simulink model "Simulation_3DOF02Testing"  (R2024a)
settings: Solver=ode4  StartTime=initial_time  StopTime=final_time  FixedStep=timestep  RelTol=1e-3
values from neighbouring files (symbols this model uses):
  alphaArray = [-30, -25, -20, -15, -10, -5, 0, 5, 10, 15, 20, 25, 30]    [Constants_3DOF.m]
  altitudeArray = [0, 1000, 2000, 3000, 4000, 5000, 6000, 7000, 8000, 9000, 10000, 15000, 20000,      25000, 30000, 35000, 40000, 45000, 50000, 55000, 60000]    [Constants_3DOF.m]
  cD_3DArray = zeros(numAoAs, numMachs, numAltitudes)    [Constants_3DOF.m]
  cL_3DArray = zeros(numAoAs, numMachs, numAltitudes)    [Constants_3DOF.m]
  flight_path_angle_0 = flight_path_angle_0 * (pi / 180)    (= 0.0523598775598)    [Constants_3DOF.m]
  heading_angle_0 = heading_angle_0 * (pi/180)    (= 0.349065850399)    [Constants_3DOF.m]
  height_0 = 35 * 10^3    (= 35000)    [Constants_3DOF.m]
  heightsList = usAtmosphere.Z    [Constants_3DOF.m]
  latitude_0 = latitude_0 * (pi/180)    (= 0.680503875353)    [Constants_3DOF.m]
  longitude_0 = longitude_0 * (pi/180)    (= -1.26396744429)    [Constants_3DOF.m]
  machArray = [0.5, 1.0, 1.5, 2.0, 2.5, 3.0, 3.5, 4.0, 4.5, 5.0, 5.5, 6.0, 6.5, 7.0, 7.5, 8.0,      8.5, 9.0, 9.5, 10.0]    [Constants_3DOF.m]
  mass = 161.5    [Constants_3DOF.m]
  omega_earth = 7.2921159 * 10^-5    (= 7.2921159e-05)    [Constants_3DOF.m]
  optimalAoA = zeros(numMachs, numAltitudes)    [Constants_3DOF.m]
  r_earth = 6371.0088 * 10^3    (= 6371008.8)    [Constants_3DOF.m]
  range_0 = 0    [Constants_3DOF.m]
  range_to_go_0 = 11112 * 10^3    (= 11112000)    [Constants_3DOF.m]
  rhoList = usAtmosphere.x_    [Constants_3DOF.m]
  speed_0 = 1500    [Constants_3DOF.m]
  temperatureList = usAtmosphere.T    [Constants_3DOF.m]
  wing_area = 0.079813    [Constants_3DOF.m]
libraries: simulink_extras x5
settings Model: Creator=641893  LastModifiedBy=641893

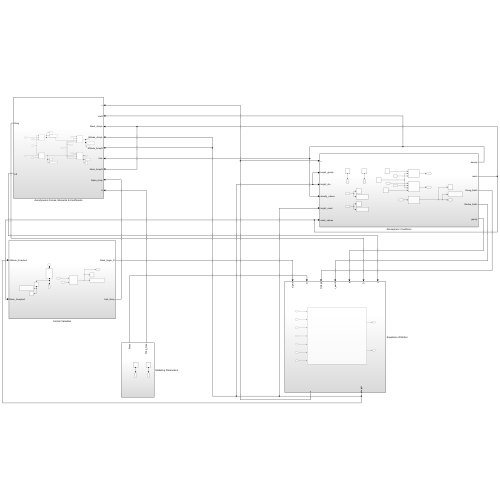
[thumbnail: Simulink's stored preview of the top-level diagram]
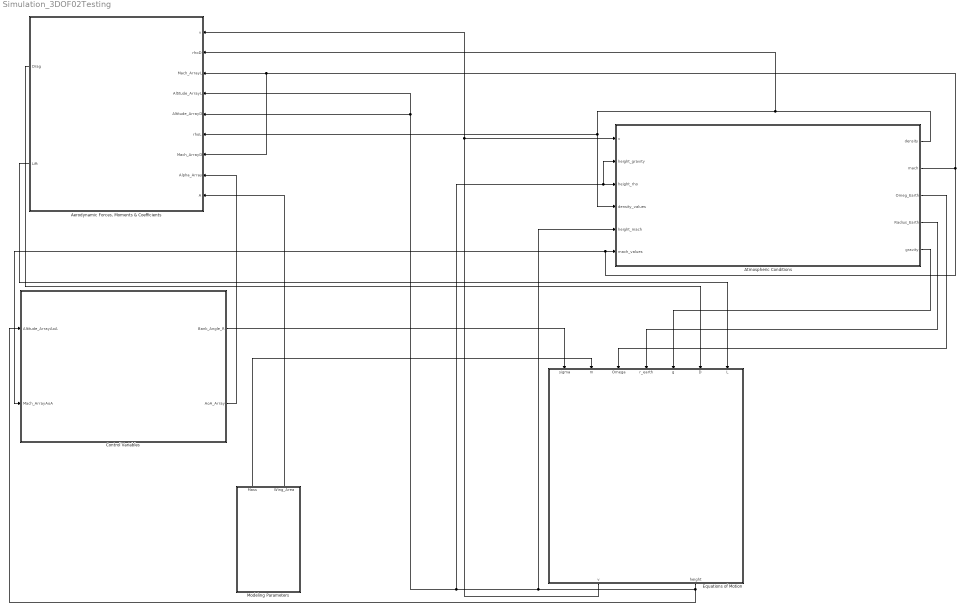
== system Simulation_3DOF02Testing ==
  "Aerodynamic Forces, Moments & Coefficients" : Subsystem
  Atmospheric Conditions : Subsystem
  Control Variables : Subsystem
  Equations of Motion : Subsystem
  Modeling Parameters : Subsystem
  wires:
  Equations of Motion/2(height) -> Atmospheric Conditions/5(height_mach), Atmospheric Conditions/3(height_rho), Atmospheric Conditions/2(height_gravity), "Aerodynamic Forces, Moments & Coefficients"/4(Altitude_ArrayL), "Aerodynamic Forces, Moments & Coefficients"/5(Altitude_ArrayD), Control Variables/1(Altitude_ArrayAoA)
  Equations of Motion/1(v) -> "Aerodynamic Forces, Moments & Coefficients"/1(v), Atmospheric Conditions/1(v)
  Atmospheric Conditions/2(mach) -> "Aerodynamic Forces, Moments & Coefficients"/3(Mach_ArrayL), "Aerodynamic Forces, Moments & Coefficients"/7(Mach_ArrayD), Atmospheric Conditions/6(mach_values), Control Variables/2(Mach_ArrayAoA)
  Atmospheric Conditions/1(density) -> Atmospheric Conditions/4(density_values), "Aerodynamic Forces, Moments & Coefficients"/6(rhoL), "Aerodynamic Forces, Moments & Coefficients"/2(rhoD)
  Atmospheric Conditions/3(Omeg_Earth) -> Equations of Motion/3(Omega)
  Atmospheric Conditions/4(Radius_Earth) -> Equations of Motion/4(r_earth)
  Atmospheric Conditions/5(gravity) -> Equations of Motion/5(g)
  "Aerodynamic Forces, Moments & Coefficients"/1(Drag) -> Equations of Motion/6(D)
  "Aerodynamic Forces, Moments & Coefficients"/2(Lift) -> Equations of Motion/7(L)
  Control Variables/1(Bank_Angle_R) -> Equations of Motion/1(sigma)
  Control Variables/2(AoA_Array) -> "Aerodynamic Forces, Moments & Coefficients"/8(Alpha_Array)
  Modeling Parameters/1(Mass) -> Equations of Motion/2(m)
  Modeling Parameters/2(Wing_Area) -> "Aerodynamic Forces, Moments & Coefficients"/9(A)

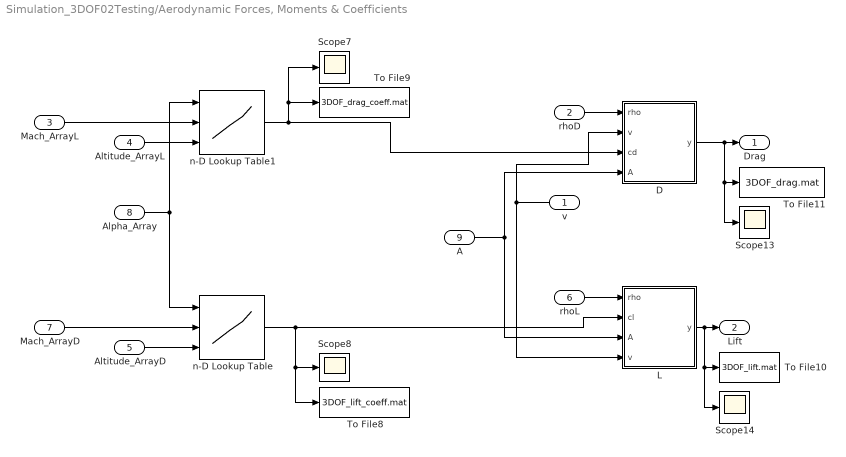
== system Simulation_3DOF02Testing/Aerodynamic Forces, Moments & Coefficients ==
  v : Inport
  rhoD : Inport  Port=2
  Mach_ArrayL : Inport  Port=3
  Altitude_ArrayL : Inport  Port=4
  Altitude_ArrayD : Inport  Port=5
  rhoL : Inport  Port=6
  Mach_ArrayD : Inport  Port=7
  Alpha_Array : Inport  Port=8
  A : Inport  Port=9
  D : MATLAB Function  TreatAsAtomicUnit=on
  L : MATLAB Function  TreatAsAtomicUnit=on
  Scope{7..8,13..14} (4 alike) : Scope
  To File10 : ToFile  Filename=3DOF_lift.mat
  To File11 : ToFile  Filename=3DOF_drag.mat
  To File8 : ToFile  Filename=3DOF_lift_coeff.mat
  To File9 : ToFile  Filename=3DOF_drag_coeff.mat
  n-D Lookup Table : Lookup_n-D  NumberOfTableDimensions=3  BreakpointsForDimension1=alphaArray  BreakpointsForDimension2=machArray  BreakpointsForDimension3=altitudeArray  IndexSearchMethod=Linear search  Table=cL_3DArray  InterpMethod=Linear Lagrange  InternalRulePriority=Speed  RndMeth=Simplest
      settings: InputPortMap=u0,u1,u2
  n-D Lookup Table1 : Lookup_n-D  NumberOfTableDimensions=3  BreakpointsForDimension1=alphaArray  BreakpointsForDimension2=machArray  BreakpointsForDimension3=altitudeArray  IndexSearchMethod=Linear search  Table=cD_3DArray  InterpMethod=Linear Lagrange  InternalRulePriority=Speed  RndMeth=Simplest
      settings: InputPortMap=u0,u1,u2
  Drag : Outport
  Lift : Outport  Port=2
  wires:
  n-D Lookup Table1/1 -> D/3(cd), Scope7/1, To File9/1
  A/1 -> L/3(A), D/4(A)
  v/1 -> D/2(v), L/4(v)
  rhoL/1 -> L/1(rho)
  Altitude_ArrayD/1 -> n-D Lookup Table/3
  n-D Lookup Table/1 -> To File8/1, Scope8/1, L/2(cl)
  Alpha_Array/1 -> n-D Lookup Table/1, n-D Lookup Table1/1
  Altitude_ArrayL/1 -> n-D Lookup Table1/3
  L/1(y) -> Scope14/1, To File10/1, Lift/1
  D/1(y) -> Scope13/1, To File11/1, Drag/1
  rhoD/1 -> D/1(rho)
  Mach_ArrayD/1 -> n-D Lookup Table/2
  Mach_ArrayL/1 -> n-D Lookup Table1/2

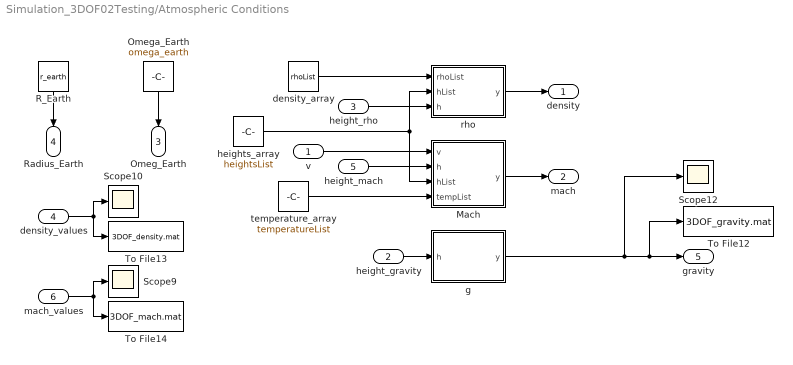
== system Simulation_3DOF02Testing/Atmospheric Conditions ==
  v : Inport
  height_gravity : Inport  Port=2
  height_rho : Inport  Port=3
  density_values : Inport  Port=4
  height_mach : Inport  Port=5
  mach_values : Inport  Port=6
  Mach : MATLAB Function  TreatAsAtomicUnit=on
  Omega_Earth : Constant  Value=omega_earth
  R_Earth : Constant  Value=r_earth
  Scope10 : Scope
  Scope12 : Scope
  Scope9 : Scope
  To File12 : ToFile  Filename=3DOF_gravity.mat
  To File13 : ToFile  Filename=3DOF_density.mat
  To File14 : ToFile  Filename=3DOF_mach.mat
  density_array : Constant  Value=rhoList
  g : MATLAB Function  TreatAsAtomicUnit=on
  heights_array : Constant  Value=heightsList
  rho : MATLAB Function  TreatAsAtomicUnit=on
  temperature_array : Constant  Value=temperatureList
  density : Outport
  mach : Outport  Port=2
  Omeg_Earth : Outport  Port=3
  Radius_Earth : Outport  Port=4
  gravity : Outport  Port=5
  wires:
  g/1(y) -> gravity/1, To File12/1, Scope12/1
  temperature_array/1 -> Mach/4(tempList)
  height_mach/1 -> Mach/2(h)
  mach_values/1 -> To File14/1, Scope9/1
  density_array/1 -> rho/1(rhoList)
  heights_array/1 -> Mach/3(hList), rho/2(hList)
  density_values/1 -> Scope10/1, To File13/1
  v/1 -> Mach/1(v)
  Mach/1(y) -> mach/1
  height_rho/1 -> rho/3(h)
  rho/1(y) -> density/1
  R_Earth/1 -> Radius_Earth/1
  Omega_Earth/1 -> Omeg_Earth/1
  height_gravity/1 -> g/1(h)

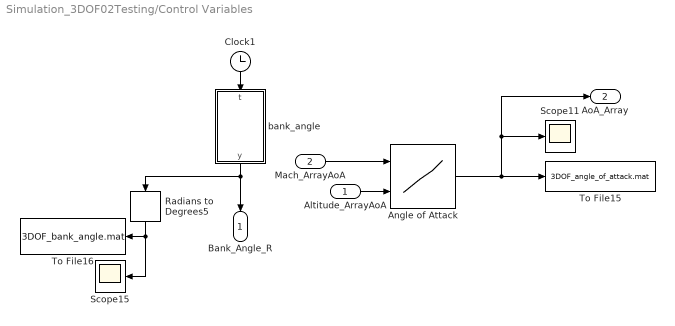
== system Simulation_3DOF02Testing/Control Variables ==
  Altitude_ArrayAoA : Inport
  Mach_ArrayAoA : Inport  Port=2
  Angle of Attack : Lookup_n-D  BreakpointsForDimension1=machArray  BreakpointsForDimension2=altitudeArray  BreakpointsForDimension3=altitudeArray  Table=optimalAoA  InterpMethod=Linear Lagrange  InternalRulePriority=Speed  RndMeth=Simplest
      settings: InputPortMap=u0,u1
  Clock1 : Clock
  Radians to Degrees5 : simulink_extras/Transformations/Radians to Degrees
  Scope11 : Scope
  Scope15 : Scope
  To File15 : ToFile  Filename=3DOF_angle_of_attack.mat
  To File16 : ToFile  Filename=3DOF_bank_angle.mat
  bank_angle : MATLAB Function  TreatAsAtomicUnit=on
  Bank_Angle_R : Outport
  AoA_Array : Outport  Port=2
  wires:
  Altitude_ArrayAoA/1 -> Angle of Attack/2
  bank_angle/1(y) -> Radians to Degrees5/1, Bank_Angle_R/1
  Angle of Attack/1 -> Scope11/1, AoA_Array/1, To File15/1
  Radians to Degrees5/1 -> Scope15/1, To File16/1
  Clock1/1 -> bank_angle/1(t)
  Mach_ArrayAoA/1 -> Angle of Attack/1

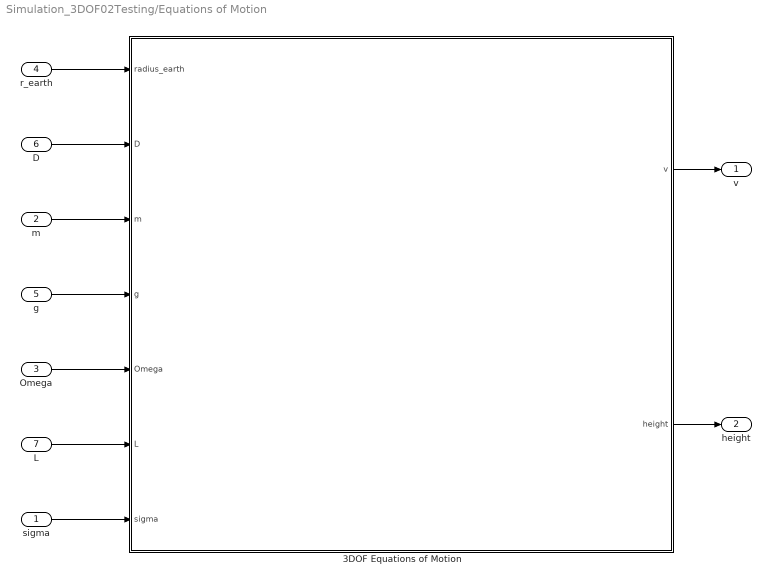
== system Simulation_3DOF02Testing/Equations of Motion ==
  sigma : Inport
  m : Inport  Port=2
  Omega : Inport  Port=3
  r_earth : Inport  Port=4
  g : Inport  Port=5
  D : Inport  Port=6
  L : Inport  Port=7
  3DOF Equations of Motion : Subsystem
  v : Outport
  height : Outport  Port=2
  wires:
  r_earth/1 -> 3DOF Equations of Motion/1(radius_earth)
  D/1 -> 3DOF Equations of Motion/2(D)
  m/1 -> 3DOF Equations of Motion/3(m)
  g/1 -> 3DOF Equations of Motion/4(g)
  Omega/1 -> 3DOF Equations of Motion/5(Omega)
  L/1 -> 3DOF Equations of Motion/6(L)
  sigma/1 -> 3DOF Equations of Motion/7(sigma)
  3DOF Equations of Motion/1(v) -> v/1
  3DOF Equations of Motion/2(height) -> height/1

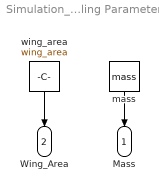
== system Simulation_3DOF02Testing/Modeling Parameters ==
  mass : Constant  Value=mass
  wing_area : Constant  Value=wing_area
  Mass : Outport
  Wing_Area : Outport  Port=2
  wires:
  wing_area/1 -> Wing_Area/1
  mass/1 -> Mass/1

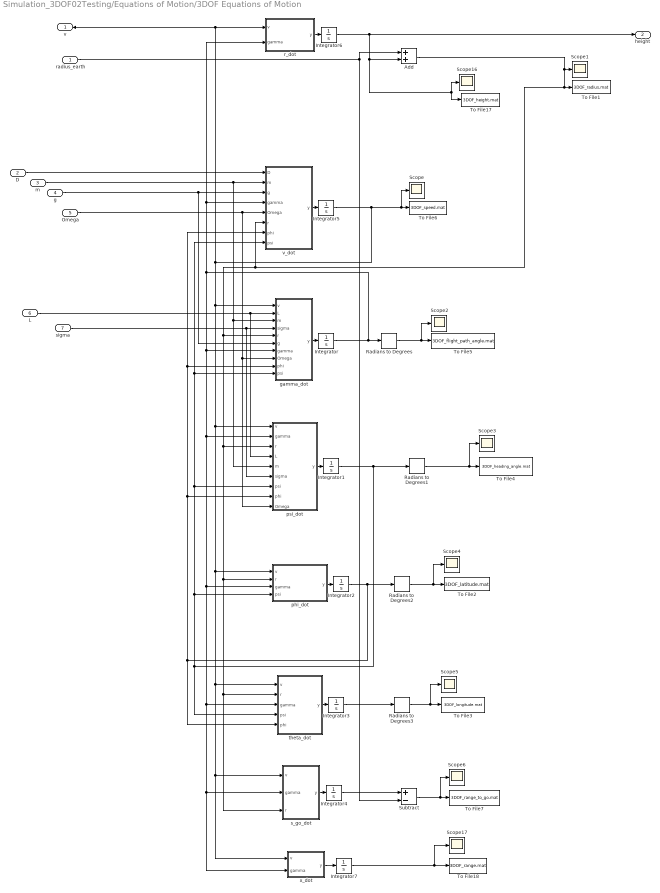
== system Simulation_3DOF02Testing/Equations of Motion/3DOF Equations of Motion ==
  radius_earth : Inport
  D : Inport  Port=2
  m : Inport  Port=3
  g : Inport  Port=4
  Omega : Inport  Port=5
  L : Inport  Port=6
  sigma : Inport  Port=7
  " x_dot" : MATLAB Function  TreatAsAtomicUnit=on
  Add : Sum
  Integrator : Integrator  InitialCondition=flight_path_angle_0
  Integrator1 : Integrator  InitialCondition=heading_angle_0
  Integrator2 : Integrator  InitialCondition=latitude_0
  Integrator3 : Integrator  InitialCondition=longitude_0
  Integrator4 : Integrator  InitialCondition=range_to_go_0
  Integrator5 : Integrator  InitialCondition=speed_0
  Integrator6 : Integrator  InitialCondition=height_0
  Integrator7 : Integrator  InitialCondition=range_0
  Radians to Degrees{,1..3} (4 alike) : simulink_extras/Transformations/Radians to Degrees
  Scope{,1..6,16..17} (9 alike) : Scope
  Subtract : Sum  Inputs=+-
  To File1 : ToFile  Filename=3DOF_radius.mat
  To File17 : ToFile  Filename=3DOF_height.mat
  To File18 : ToFile  Filename=3DOF_range.mat
  To File2 : ToFile  Filename=3DOF_latitude.mat
  To File3 : ToFile  Filename=3DOF_longitude.mat
  To File4 : ToFile  Filename=3DOF_heading_angle.mat
  To File5 : ToFile  Filename=3DOF_flight_path_angle.mat
  To File6 : ToFile  Filename=3DOF_speed.mat
  To File7 : ToFile  Filename=3DOF_range_to_go.mat
  gamma_dot : MATLAB Function  TreatAsAtomicUnit=on
  phi_dot : MATLAB Function  TreatAsAtomicUnit=on
  psi_dot : MATLAB Function  TreatAsAtomicUnit=on
  r_dot : MATLAB Function  TreatAsAtomicUnit=on
  s_go_dot : MATLAB Function  TreatAsAtomicUnit=on
  theta_dot : MATLAB Function  TreatAsAtomicUnit=on
  v_dot : MATLAB Function  TreatAsAtomicUnit=on
  v : Outport
  height : Outport  Port=2
  wires:
  radius_earth/1 -> Add/1, Subtract/2
  Radians to Degrees3/1 -> To File3/1, Scope5/1
  Integrator4/1 -> Subtract/1
  Integrator7/1 -> To File18/1, Scope17/1
  Integrator5/1 -> " x_dot"/1(v), s_go_dot/1(v), theta_dot/1(v), phi_dot/1(v), psi_dot/1(v), gamma_dot/1(v), v/1, r_dot/1(v), Scope/1, To File6/1
  Integrator1/1 -> phi_dot/4(psi), psi_dot/7(psi), gamma_dot/10(psi), v_dot/8(psi), theta_dot/4(psi), Radians to Degrees1/1
  Add/1 -> v_dot/6(r), s_go_dot/3(r), theta_dot/2(r), phi_dot/2(r), psi_dot/3(r), gamma_dot/5(r), To File1/1, Scope1/1
  Integrator2/1 -> theta_dot/5(phi), psi_dot/8(phi), gamma_dot/9(phi), v_dot/7(phi), Radians to Degrees2/1
  Integrator6/1 -> height/1, To File17/1, Scope16/1, Add/2
  Integrator/1 -> " x_dot"/2(gamma), s_go_dot/2(gamma), theta_dot/3(gamma), phi_dot/3(gamma), psi_dot/2(gamma), gamma_dot/7(gamma), r_dot/2(gamma), v_dot/4(gamma), Radians to Degrees/1
  m/1 -> psi_dot/5(m), gamma_dot/3(m), v_dot/2(m)
  Integrator3/1 -> Radians to Degrees3/1
  " x_dot"/1(y) -> Integrator7/1
  sigma/1 -> psi_dot/6(sigma), gamma_dot/4(sigma)
  g/1 -> gamma_dot/6(g), v_dot/3(g)
  psi_dot/1(y) -> Integrator1/1
  v_dot/1(y) -> Integrator5/1
  r_dot/1(y) -> Integrator6/1
  Radians to Degrees2/1 -> To File2/1, Scope4/1
  L/1 -> psi_dot/4(L), gamma_dot/2(L)
  s_go_dot/1(y) -> Integrator4/1
  theta_dot/1(y) -> Integrator3/1
  phi_dot/1(y) -> Integrator2/1
  gamma_dot/1(y) -> Integrator/1
  Radians to Degrees/1 -> To File5/1, Scope2/1
  Omega/1 -> v_dot/5(Omega), psi_dot/9(Omega), gamma_dot/8(Omega)
  Subtract/1 -> To File7/1, Scope6/1
  Radians to Degrees1/1 -> Scope3/1, To File4/1
  D/1 -> v_dot/1(D)

== matlab function Simulation_3DOF02Testing/Aerodynamic Forces, Moments & Coefficients/D ==
  data: rho input; y output; v input; cd input; A input
function y = fcn(rho, v, cd, A)

y = 0.5 * rho * v^2 * A * cd;

== matlab function Simulation_3DOF02Testing/Atmospheric Conditions/g ==
  data: y output; h input
function y = fcn(h)
mu_earth = 3.96272 * 10^14;
rE = 6378140;
y = mu_earth / (rE + h)^2;

== matlab function Simulation_3DOF02Testing/Atmospheric Conditions/rho ==
  data: rhoList input; hList input; h input; y output
function y = fcn(rhoList, hList,h)

h = h / 10^3;

if h >= 0
    density = interp1(hList, rhoList, h);
else
    density = 0;
end


y = density;

== matlab function Simulation_3DOF02Testing/Equations of Motion/3DOF Equations of Motion/ x_dot ==
  data: v input; y output; gamma input
function y = fcn(v, gamma)

y = v * cos(gamma);

== matlab function Simulation_3DOF02Testing/Atmospheric Conditions/Mach ==
  data: v input; y output; h input; hList input; tempList input
function y = fcn(v, h, hList, tempList)

gamma = 1.4;
R = 287.05;

h = h / 10^3;

if h >= 0
    temp = interp1(hList, tempList, h);
    a = sqrt(gamma * R * temp);
    y = v/a;
else
    temp = 0;
    y = 0;
end

== matlab function Simulation_3DOF02Testing/Control Variables/bank_angle ==
  data: t input; y output
function y = fcn(t)

sigma = 0;
sigma = sigma * pi / 180;

y = sigma;

== matlab function Simulation_3DOF02Testing/Equations of Motion/3DOF Equations of Motion/phi_dot ==
  data: v input; y output; r input; gamma input; psi input
function y = fcn(v, r, gamma, psi)

y = (v / r) * cos(gamma) * sin(psi);

== matlab function Simulation_3DOF02Testing/Equations of Motion/3DOF Equations of Motion/r_dot ==
  data: v input; y output; gamma input
function y = fcn(v, gamma)

y = v * sin(gamma);

== matlab function Simulation_3DOF02Testing/Equations of Motion/3DOF Equations of Motion/theta_dot ==
  data: v input; y output; r input; gamma input; psi input; phi input
function y = fcn(v, r, gamma, psi, phi)

y = (v * cos(gamma) * cos(psi) ) / (r * cos(phi) );

== matlab function Simulation_3DOF02Testing/Equations of Motion/3DOF Equations of Motion/v_dot ==
  data: D input; y output; m input; g input; gamma input; Omega input; r input; phi input; psi input
function y = fcn(D, m, g, gamma, Omega, r, phi, psi)

y = -(D / m) - g * sin(gamma) + Omega^2 * r * cos(phi) * ( sin(gamma) * cos(phi) - cos(gamma) * sin(phi) * cos(psi) );

== matlab function Simulation_3DOF02Testing/Equations of Motion/3DOF Equations of Motion/gamma_dot ==
  data: v input; y output; L input; m input; sigma input; r input; g input; gamma input; Omega input; phi input; psi input
function y = fcn(v, L, m, sigma, r, g, gamma, Omega, phi, psi)

y = (1/v) * ( (L / m) * cos(sigma) + (( v^2 / r) - g) * cos(gamma) + 2 * Omega * v * cos(phi) * sin(psi) + Omega^2 * r * cos(phi) * ( cos(gamma) * cos(phi) - sin(gamma) * sin(phi) * cos(psi) ) );

== matlab function Simulation_3DOF02Testing/Equations of Motion/3DOF Equations of Motion/psi_dot ==
  data: v input; y output; gamma input; r input; L input; m input; sigma input; psi input; phi input; Omega input
function y = fcn(v, gamma, r, L, m, sigma, psi, phi, Omega)

y = (1 / v) * ( (L / (m * cos(gamma))) * sin(sigma) + (v^2 /  r) * cos(gamma) * sin(psi) * tan(phi) - 2 * Omega * v * (tan(gamma) * cos(psi) * cos(phi) - sin(phi) ) + (Omega^2 * r / cos(gamma)) * sin(psi) * sin(phi) * cos(phi) );

== matlab function Simulation_3DOF02Testing/Equations of Motion/3DOF Equations of Motion/s_go_dot ==
  data: v input; y output; gamma input; r input
function y = fcn(v, gamma, r)
rE = 6378140;
y = -v * cos(gamma) * rE / r;

== matlab function Simulation_3DOF02Testing/Aerodynamic Forces, Moments & Coefficients/L ==
  data: rho input; y output; cl input; A input; v input
function y = fcn(rho, cl, A, v)

y = 0.5 * rho * v^2 * A * cl;
